simulink model "UAM_Status"  (R2024b)
settings: Solver=VariableStepAuto  StartTime=0.0  StopTime=10.0  RelTol=1e-3
libraries: mspfiltlib x1, robotcorelib x1
settings Model: Creator=admin  LastModifiedBy=USER

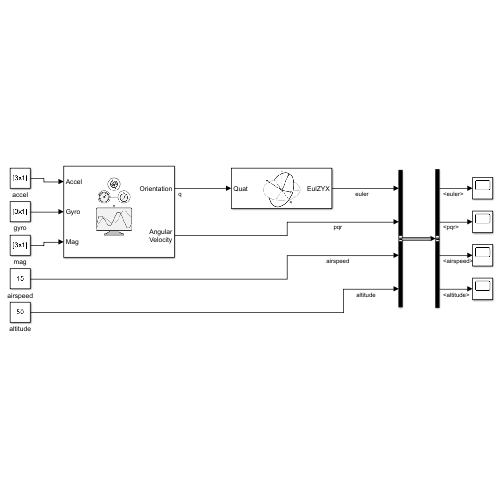
[thumbnail: Simulink's stored preview of the top-level diagram]
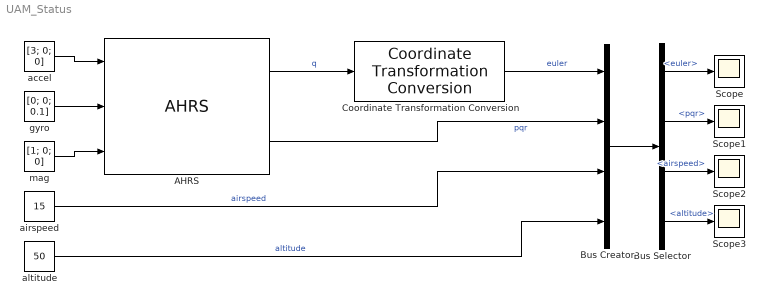
== system UAM_Status ==
  AHRS : mspfiltlib/AHRS  DispRefFrame=NED  DecimationFactor=1  InitialProcessNoise=ahrsfilter.defaultProcessNoise  OrientationFormat=quaternion  SimulateUsing=Interpreted execution  AccelerometerNoise=0.0001924722  GyroscopeNoise=9.1385e-5  MagnetometerNoise=0.1  GyroscopeDriftNoise=3.0462e-13  LinearAccelerationNoise=0.0096236100000000012  MagneticDisturbanceNoise=0.5  LinearAccelerationDecayFactor=0.5  MagneticDisturbanceDecayFactor=0.5  ExpectedMagneticFieldStrength=50
  Bus Creator : BusCreator  Inputs=4
  Bus Selector : BusSelector  OutputSignals=euler,pqr,airspeed,altitude
  Coordinate Transformation Conversion : robotcorelib/Coordinate Transformation Conversion  InputRepresentation=Quaternion  InputEulerSequence=ZYX  ShowTrVecInputPort=on  OutputRepresentation=Euler Angles  OutputEulerSequence=ZYX  ShowTrVecOutputPort=on  SimulateUsing=Interpreted execution
      settings: LibrarySourceBlock=navlib/Utilities/Coordinate Transformation Conversion
  Scope{,1..3} (4 alike) : Scope
  accel : Constant  Value=[3; 0; 0]  VectorParams1D=off
  airspeed : Constant  Value=15  VectorParams1D=off
  altitude : Constant  Value=50  VectorParams1D=off
  gyro : Constant  Value=[0; 0; 0.1]  VectorParams1D=off
  mag : Constant  Value=[1; 0; 0]  VectorParams1D=off
  wires:
  gyro/1 -> AHRS/2
  accel/1 -> AHRS/1
  mag/1 -> AHRS/3
  AHRS/1 -> Coordinate Transformation Conversion/1  "q"
  Coordinate Transformation Conversion/1 -> Bus Creator/1  "euler"
  AHRS/2 -> Bus Creator/2  "pqr"
  airspeed/1 -> Bus Creator/3  "airspeed"
  altitude/1 -> Bus Creator/4  "altitude"
  Bus Creator/1 -> Bus Selector/1
  Bus Selector/1 -> Scope/1  "<euler>"
  Bus Selector/2 -> Scope1/1  "<pqr>"
  Bus Selector/3 -> Scope2/1  "<airspeed>"
  Bus Selector/4 -> Scope3/1  "<altitude>"
